simulink model "raibert_controller_1_2"  (R2018b)
settings: Solver=FixedStepDiscrete  StartTime=0.0  StopTime=inf  FixedStep=sample_time  RelTol=1e-3
InitFcn:
  | raibert_controller_params_1_2
  | warning off all
values from neighbouring files (symbols this model uses):
  sample_time = 1/sample_freq    (= 0.001)    [simulation_params.m]
undefined symbols (not defined in the file or in its folder): ctrl, Discrete, initial_dx_estimate, initial_dy_estimate, initial_dz_estimate, initial_z_estimate, Time
libraries: simulink x30, ctrlSharedLib x7
(part 2 of 4)

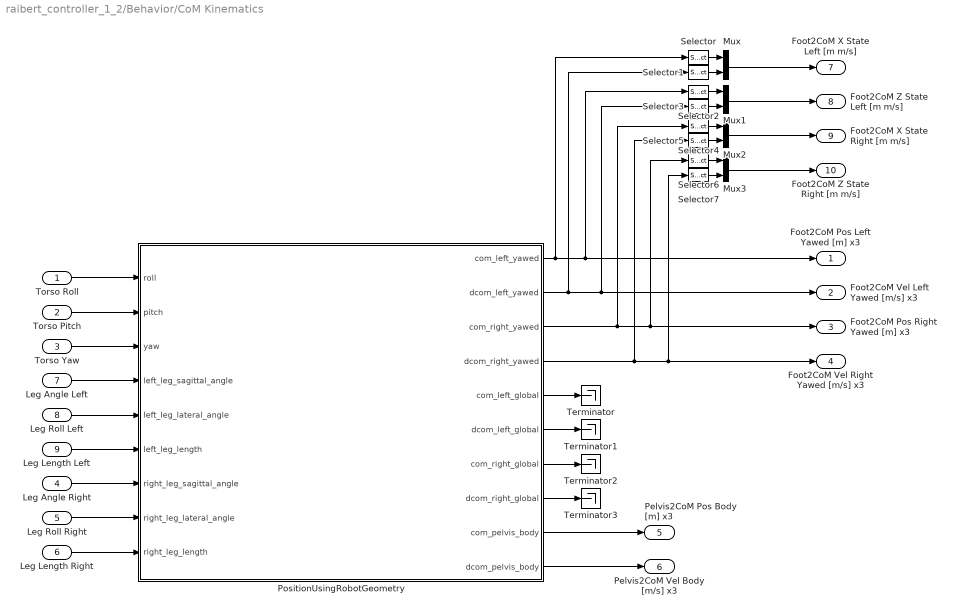
== system raibert_controller_1_2/Behavior/CoM Kinematics ==
  Torso Roll : Inport
  Torso Pitch : Inport  Port=2
  Torso Yaw : Inport  Port=3
  Leg Angle Right : Inport  Port=4
  Leg Roll Right : Inport  Port=5
  Leg Length Right : Inport  Port=6
  Leg Angle Left : Inport  Port=7
  Leg Roll Left : Inport  Port=8
  Leg Length Left : Inport  Port=9
  Mux{,1..3} (4 alike) : Mux  Inputs=2
  PositionUsingRobotGeometry : MATLAB Function  TreatAsAtomicUnit=on
  Selector{,1,4..5} (4 alike) : Selector  InputPortWidth=3  IndexOptions=Index vector (dialog)  Indices=[1]  OutputSizes=1
  Selector{2..3,6..7} (4 alike) : Selector  InputPortWidth=3  IndexOptions=Index vector (dialog)  Indices=[3]  OutputSizes=1
  Terminator{,1..3} (4 alike) : Terminator
  Foot2CoM Pos Left Yawed [m] x3 : Outport
  Foot2CoM Vel Left Yawed [m/s] x3 : Outport  Port=2
  Foot2CoM Pos Right Yawed [m] x3 : Outport  Port=3
  Foot2CoM Vel Right Yawed [m/s] x3 : Outport  Port=4
  Pelvis2CoM Pos Body [m] x3 : Outport  Port=5
  Pelvis2CoM Vel Body [m/s] x3 : Outport  Port=6
  Foot2CoM X State Left [m m/s] : Outport  Port=7
  Foot2CoM Z State Left [m m/s] : Outport  Port=8
  Foot2CoM X State Right [m m/s] : Outport  Port=9
  Foot2CoM Z State Right [m m/s] : Outport  Port=10
  wires:
  Leg Angle Left/1 -> PositionUsingRobotGeometry/4(left_leg_sagittal_angle)
  Leg Roll Left/1 -> PositionUsingRobotGeometry/5(left_leg_lateral_angle)
  Leg Length Left/1 -> PositionUsingRobotGeometry/6(left_leg_length)
  Leg Angle Right/1 -> PositionUsingRobotGeometry/7(right_leg_sagittal_angle)
  Leg Roll Right/1 -> PositionUsingRobotGeometry/8(right_leg_lateral_angle)
  Leg Length Right/1 -> PositionUsingRobotGeometry/9(right_leg_length)
  Torso Roll/1 -> PositionUsingRobotGeometry/1(roll)
  Torso Yaw/1 -> PositionUsingRobotGeometry/3(yaw)
  Torso Pitch/1 -> PositionUsingRobotGeometry/2(pitch)
  PositionUsingRobotGeometry/3(com_right_yawed) -> Selector4/1, Selector6/1, Foot2CoM Pos Right Yawed [m] x3/1
  PositionUsingRobotGeometry/4(dcom_right_yawed) -> Selector5/1, Selector7/1, Foot2CoM Vel Right Yawed [m/s] x3/1
  PositionUsingRobotGeometry/1(com_left_yawed) -> Foot2CoM Pos Left Yawed [m] x3/1, Selector2/1, Selector/1
  PositionUsingRobotGeometry/2(dcom_left_yawed) -> Selector3/1, Foot2CoM Vel Left Yawed [m/s] x3/1, Selector1/1
  PositionUsingRobotGeometry/10(dcom_pelvis_body) -> Pelvis2CoM Vel Body [m/s] x3/1
  PositionUsingRobotGeometry/9(com_pelvis_body) -> Pelvis2CoM Pos Body [m] x3/1
  PositionUsingRobotGeometry/5(com_left_global) -> Terminator/1
  PositionUsingRobotGeometry/6(dcom_left_global) -> Terminator1/1
  PositionUsingRobotGeometry/7(com_right_global) -> Terminator2/1
  PositionUsingRobotGeometry/8(dcom_right_global) -> Terminator3/1
  Selector/1 -> Mux/1
  Selector1/1 -> Mux/2
  Mux/1 -> Foot2CoM X State Left [m m/s]/1
  Selector3/1 -> Mux1/2
  Selector2/1 -> Mux1/1
  Mux1/1 -> Foot2CoM Z State Left [m m/s]/1
  Mux3/1 -> Foot2CoM Z State Right [m m/s]/1
  Selector6/1 -> Mux3/1
  Selector7/1 -> Mux3/2
  Mux2/1 -> Foot2CoM X State Right [m m/s]/1
  Selector5/1 -> Mux2/2
  Selector4/1 -> Mux2/1

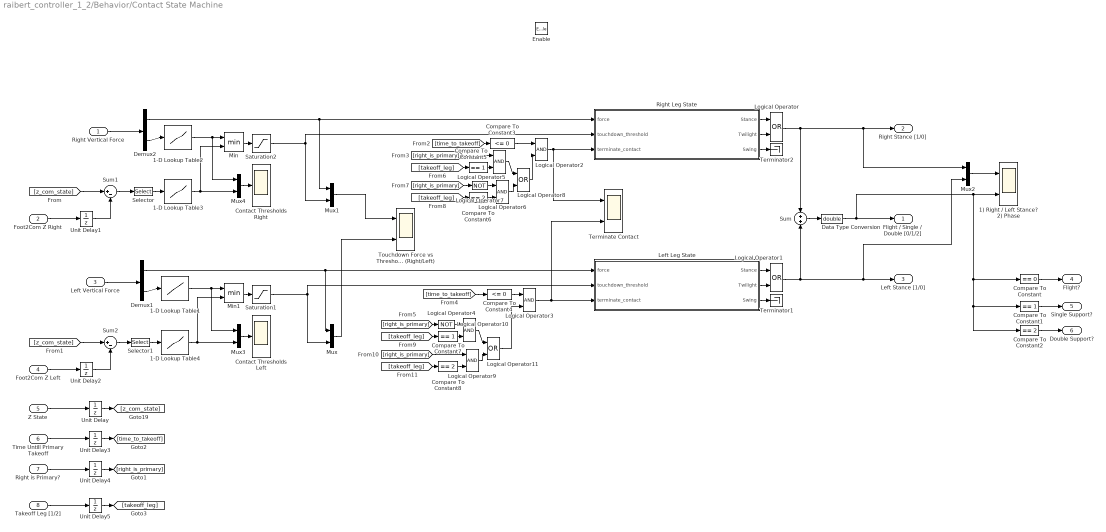
== system raibert_controller_1_2/Behavior/Contact State Machine ==
  Right Vertical Force : Inport
  Foot2Com Z Right : Inport  Port=2
  Left Vertical Force : Inport  Port=3
  Foot2Com Z Left : Inport  Port=4
  Z State : Inport  Port=5
  Time Untill Primary Takeoff : Inport  Port=6
  Right is Primary? : Inport  Port=7
  Takeoff Leg [1/2] : Inport  Port=8
  Enable : EnablePort  StatesWhenEnabling=reset
  1) Right / Left Stance? 2) Phase : Scope  NumInputPorts=2
  1-D Lookup Table1 : Lookup_n-D  NumberOfTableDimensions=1  BreakpointsForDimension1=[0, ctrl.touchdown_force_rate_hi]  Table=[ctrl.touchdown_threshold_hi, ctrl.touchdown_threshold_lo]  InternalRulePriority=Speed  RndMeth=Simplest  InputSameDT=on
  1-D Lookup Table2 : Lookup_n-D  NumberOfTableDimensions=1  BreakpointsForDimension1=[0, ctrl.touchdown_force_rate_hi]  Table=[ctrl.touchdown_threshold_hi, ctrl.touchdown_threshold_lo]  InternalRulePriority=Speed  RndMeth=Simplest  InputSameDT=on
  1-D Lookup Table3 : Lookup_n-D  NumberOfTableDimensions=1  BreakpointsForDimension1=[0, ctrl.touchdown_dist_hi]  Table=[ctrl.touchdown_threshold_lo, ctrl.touchdown_threshold_hi]  InternalRulePriority=Speed  RndMeth=Simplest  InputSameDT=on
  1-D Lookup Table4 : Lookup_n-D  NumberOfTableDimensions=1  BreakpointsForDimension1=[0, ctrl.touchdown_dist_hi]  Table=[ctrl.touchdown_threshold_lo, ctrl.touchdown_threshold_hi]  InternalRulePriority=Speed  RndMeth=Simplest  InputSameDT=on
  Compare To Constant : simulink/Logic and Bit Operations/Compare To Constant  relop===  const=0  OutDataTypeStr=boolean
  Compare To Constant1 : simulink/Logic and Bit Operations/Compare To Constant  relop===  const=1  OutDataTypeStr=boolean
  Compare To Constant2 : simulink/Logic and Bit Operations/Compare To Constant  relop===  const=2  OutDataTypeStr=boolean
  Compare To Constant3 : simulink/Logic and Bit Operations/Compare To Constant  relop=<=  const=0  OutDataTypeStr=boolean
  Compare To Constant4 : simulink/Logic and Bit Operations/Compare To Constant  relop=<=  const=0  OutDataTypeStr=boolean
  Compare To Constant5 : simulink/Logic and Bit Operations/Compare To Constant  relop===  const=1  OutDataTypeStr=boolean
  Compare To Constant6 : simulink/Logic and Bit Operations/Compare To Constant  relop===  const=2  OutDataTypeStr=boolean
  Compare To Constant7 : simulink/Logic and Bit Operations/Compare To Constant  relop===  const=1  OutDataTypeStr=boolean
  Compare To Constant8 : simulink/Logic and Bit Operations/Compare To Constant  relop===  const=2  OutDataTypeStr=boolean
  Contact Thresholds Left : Scope
  Contact Thresholds Right : Scope
  Data Type Conversion : DataTypeConversion  OutDataTypeStr=double
  Demux1 : Demux  Outputs=2
  Demux2 : Demux  Outputs=2
  Left Leg State : State Transition Table  TreatAsAtomicUnit=on
  Logical Operator{,1,8,11} (4 alike) : Logic  Operator=OR  AllPortsSameDT=off  OutDataTypeStr=boolean
  Logical Operator10 : Logic  Operator=NOT  AllPortsSameDT=off  OutDataTypeStr=boolean
  Logical Operator{2..6,9} (6 alike) : Logic  AllPortsSameDT=off  OutDataTypeStr=boolean
  Logical Operator7 : Logic  Operator=NOT  AllPortsSameDT=off  OutDataTypeStr=boolean
  Min : MinMax  Inputs=2
  Min1 : MinMax  Inputs=2
  Mux{,1..4} (5 alike) : Mux  Inputs=2
  Right Leg State : State Transition Table  TreatAsAtomicUnit=on
  Saturation1 : Saturate  UpperLimit=ctrl.touchdown_threshold_hi  LowerLimit=ctrl.touchdown_threshold_lo
  Saturation2 : Saturate  UpperLimit=ctrl.touchdown_threshold_hi  LowerLimit=ctrl.touchdown_threshold_lo
  Selector : Selector  InputPortWidth=2  IndexOptions=Index vector (dialog)  Indices=[1]  OutputSizes=1
  Selector1 : Selector  InputPortWidth=2  IndexOptions=Index vector (dialog)  Indices=[1]  OutputSizes=1
  Sum : Sum  Inputs=+|+
  Sum1 : Sum  Inputs=|+-
  Sum2 : Sum  Inputs=|+-
  Terminate Contact : Scope  NumInputPorts=2
  Terminator1 : Terminator
  Terminator2 : Terminator
  Touchdown Force vs Threshold (Right/Left) : Scope  NumInputPorts=2
  Unit Delay{,1..5} (6 alike) : UnitDelay  SampleTime=-1
  Flight / Single / Double [0/1/2] : Outport  InitialOutput=0
  Right Stance [1/0] : Outport  Port=2  InitialOutput=0
  Left Stance [1/0] : Outport  Port=3  InitialOutput=0
  Flight? : Outport  Port=4  InitialOutput=true
  Single Support? : Outport  Port=5  InitialOutput=false
  Double Support? : Outport  Port=6  InitialOutput=false
  wires:
  Left Leg State/3(" Swing") -> Terminator1/1
  Logical Operator/1 -> Sum/1, Mux2/1, Right Stance [1/0]/1
  Left Vertical Force/1 -> Demux1/1
  Demux1/2 -> 1-D Lookup Table1/1
  Demux1/1 -> Left Leg State/1(force), Mux/1
  Saturation1/1 -> Mux/2, Left Leg State/2(touchdown_threshold)
  Logical Operator1/1 -> Sum/2, Mux2/2, Left Stance [1/0]/1
  Mux/1 -> Touchdown Force vs Threshold (Right/Left)/2
  Mux1/1 -> Touchdown Force vs Threshold (Right/Left)/1
  Saturation2/1 -> Mux1/2, Right Leg State/2(touchdown_threshold)
  Demux2/1 -> Right Leg State/1(force), Mux1/1
  Demux2/2 -> 1-D Lookup Table2/1
  Right Vertical Force/1 -> Demux2/1
  Min/1 -> Saturation2/1
  Mux2/1 -> 1) Right / Left Stance? 2) Phase/1
  Sum/1 -> Data Type Conversion/1
  Compare To Constant/1 -> Flight?/1
  Compare To Constant1/1 -> Single Support?/1
  Compare To Constant2/1 -> Double Support?/1
  Data Type Conversion/1 -> Compare To Constant2/1, Compare To Constant1/1, Compare To Constant/1, 1) Right / Left Stance? 2) Phase/2, Flight / Single / Double [0/1/2]/1
  Right Leg State/3(" Swing") -> Terminator2/1
  Right Leg State/2(" Twilight") -> Logical Operator/2
  Right Leg State/1(" Stance") -> Logical Operator/1
  Left Leg State/1(" Stance") -> Logical Operator1/1
  Left Leg State/2(" Twilight") -> Logical Operator1/2
  Z State/1 -> Unit Delay/1
  [z_com_state] -> Sum1/1
  Foot2Com Z Right/1 -> Unit Delay1/1
  Foot2Com Z Left/1 -> Unit Delay2/1
  [z_com_state] -> Sum2/1
  Sum1/1 -> Selector/1
  1-D Lookup Table2/1 -> Mux4/1, Min/1
  1-D Lookup Table3/1 -> Mux4/2, Min/2
  Sum2/1 -> Selector1/1
  1-D Lookup Table1/1 -> Mux3/1, Min1/1
  1-D Lookup Table4/1 -> Min1/2, Mux3/2
  Min1/1 -> Saturation1/1
  Mux3/1 -> Contact Thresholds Left/1
  Mux4/1 -> Contact Thresholds Right/1
  Selector/1 -> 1-D Lookup Table3/1
  Selector1/1 -> 1-D Lookup Table4/1
  Unit Delay/1 -> [z_com_state]
  Unit Delay1/1 -> Sum1/2
  Unit Delay2/1 -> Sum2/2
  Right is Primary?/1 -> Unit Delay4/1
  Time Untill Primary Takeoff/1 -> Unit Delay3/1
  [time_to_takeoff] -> Compare To Constant3/1
  Compare To Constant3/1 -> Logical Operator2/1
  [right_is_primary] -> Logical Operator5/1
  Logical Operator2/1 -> Terminate Contact/1, Right Leg State/3(terminate_contact)
  Unit Delay3/1 -> [time_to_takeoff]
  Unit Delay4/1 -> [right_is_primary]
  Compare To Constant4/1 -> Logical Operator3/1
  [time_to_takeoff] -> Compare To Constant4/1
  Logical Operator3/1 -> Left Leg State/3(terminate_contact), Terminate Contact/2
  Takeoff Leg [1/2]/1 -> Unit Delay5/1
  Unit Delay5/1 -> [takeoff_leg]
  [takeoff_leg] -> Compare To Constant5/1
  Compare To Constant5/1 -> Logical Operator5/2
  Compare To Constant6/1 -> Logical Operator6/2
  [takeoff_leg] -> Compare To Constant6/1
  [right_is_primary] -> Logical Operator7/1
  Logical Operator7/1 -> Logical Operator6/1
  Logical Operator5/1 -> Logical Operator8/1
  Logical Operator6/1 -> Logical Operator8/2
  Logical Operator8/1 -> Logical Operator2/2
  [right_is_primary] -> Logical Operator10/1
  Compare To Constant7/1 -> Logical Operator4/2
  Logical Operator4/1 -> Logical Operator11/1
  [takeoff_leg] -> Compare To Constant7/1
  Logical Operator9/1 -> Logical Operator11/2
  [right_is_primary] -> Logical Operator9/1
  Compare To Constant8/1 -> Logical Operator9/2
  [takeoff_leg] -> Compare To Constant8/1
  Logical Operator10/1 -> Logical Operator4/1
  Logical Operator11/1 -> Logical Operator3/2

== system raibert_controller_1_2/Behavior/Filter Gyro Velocities ==
  raw dq : Inport
  Demux : Demux  Outputs=3
  Demux1 : Demux  Outputs=3
  Fourbar : Selector  InputPortWidth=13  IndexOptions=Index vector (dialog)  Indices=[1 2 3 4 5 6 7 8]  OutputSizes=1
  IMU Two Pole Filter : DiscreteTransferFcn  Numerator=[ctrl.A_imu 0 0]  Denominator=[1 ctrl.B1_imu ctrl.B2_imu]  SampleTime=sample_time
  Lateral : Selector  InputPortWidth=13  IndexOptions=Index vector (dialog)  Indices=[9 10]  OutputSizes=1
  Mux : Mux  Inputs=3
  Mux25 : Mux  Inputs=2
  Mux26 : Mux  Inputs=2
  Mux27 : Mux  Inputs=2
  Torso Orientation : Selector  InputPortWidth=13  IndexOptions=Index vector (dialog)  Indices=[11 12 13]  OutputSizes=1
  Torso Orientation Filter : Scope  NumInputPorts=3
  filtered dq : Outport
  wires:
  Fourbar/1 -> Mux/1
  IMU Two Pole Filter/1 -> Demux1/1, Mux/3
  Mux/1 -> filtered dq/1
  raw dq/1 -> Fourbar/1, Torso Orientation/1, Lateral/1
  Torso Orientation/1 -> Demux/1, IMU Two Pole Filter/1
  Lateral/1 -> Mux/2
  Mux25/1 -> Torso Orientation Filter/1
  Mux27/1 -> Torso Orientation Filter/3
  Mux26/1 -> Torso Orientation Filter/2
  Demux/1 -> Mux25/1
  Demux/2 -> Mux26/1
  Demux/3 -> Mux27/1
  Demux1/1 -> Mux25/2
  Demux1/2 -> Mux26/2
  Demux1/3 -> Mux27/2

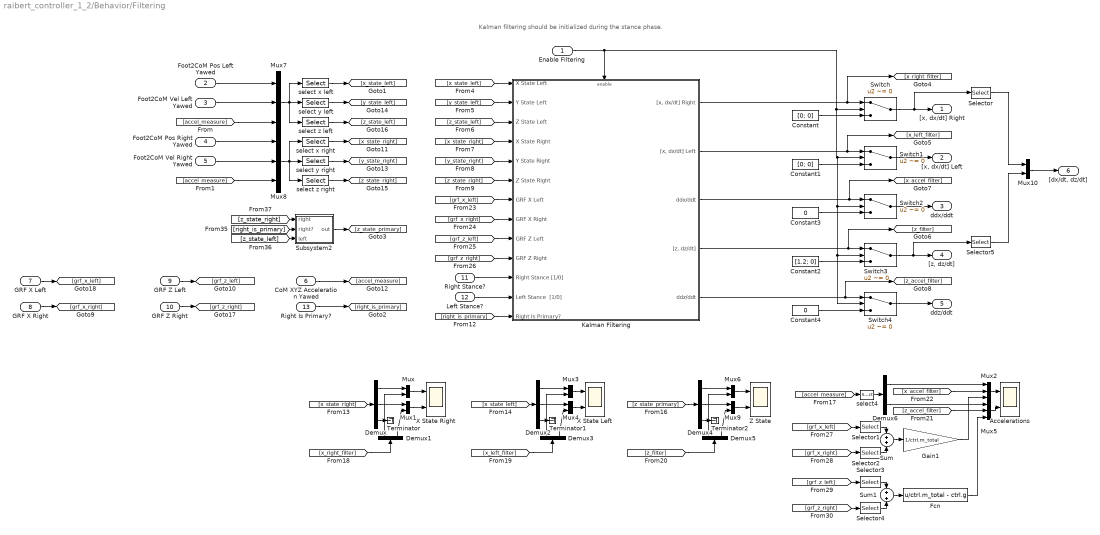
== system raibert_controller_1_2/Behavior/Filtering ==
  note: Kalman filtering should be initialized during the stance phase.
  Enable Filtering : Inport
  Foot2CoM Pos Left Yawed : Inport  Port=2
  Foot2CoM Vel Left Yawed : Inport  Port=3
  Foot2CoM Pos Right Yawed : Inport  Port=4
  Foot2CoM Vel Right Yawed : Inport  Port=5
  CoM XYZ Acceleration Yawed : Inport  Port=6
  GRF X Left : Inport  Port=7
  GRF X Right : Inport  Port=8
  GRF Z Left : Inport  Port=9
  GRF Z Right : Inport  Port=10
  Right Stance? : Inport  Port=11
  Left Stance? : Inport  Port=12
  Right Is Primary? : Inport  Port=13
  Accelerations : Scope  NumInputPorts=2
  Constant : Constant  Value=[0; 0]
  Constant1 : Constant  Value=[0; 0]
  Constant2 : Constant  Value=[1.2; 0]
  Constant3 : Constant  Value=0
  Constant4 : Constant  Value=0
  Demux : Demux  Outputs=3
  Demux{1,3,5..6} (4 alike) : Demux  Outputs=2
  Demux2 : Demux  Outputs=3
  Demux4 : Demux  Outputs=3
  Fcn : Fcn  Expr=u/ctrl.m_total - ctrl.g
  Gain1 : Gain  Gain=1/ctrl.m_total
  Kalman Filtering : Subsystem
  Mux{,1,3..4,6,9..10} (7 alike) : Mux  Inputs=2
  Mux{2,5,7..8} (4 alike) : Mux  Inputs=3
  Selector : Selector  InputPortWidth=2  IndexOptions=Index vector (dialog)  Indices=[2]  OutputSizes=1
  Selector{1..4} (4 alike) : Selector  InputPortWidth=2  IndexOptions=Index vector (dialog)  Indices=[1]  OutputSizes=1
  Selector5 : Selector  InputPortWidth=2  IndexOptions=Index vector (dialog)  Indices=[2]  OutputSizes=1
  Subsystem2 : Subsystem
  Sum : Sum  Inputs=+|+
  Sum1 : Sum  Inputs=+|+
  Switch{,1..4} (5 alike) : Switch  Criteria=u2 ~= 0
  Terminator : Terminator
  Terminator1 : Terminator
  Terminator2 : Terminator
  X State Left : Scope  NumInputPorts=2
  X State Right : Scope  NumInputPorts=2
  Z State : Scope  NumInputPorts=2
  select x left : Selector  InputPortWidth=9  IndexOptions=Index vector (dialog)  Indices=[1 4 7]  OutputSizes=1
  select x right : Selector  InputPortWidth=9  IndexOptions=Index vector (dialog)  Indices=[1 4 7]  OutputSizes=1
  select y left : Selector  InputPortWidth=9  IndexOptions=Index vector (dialog)  Indices=[2 5 8]  OutputSizes=1
  select y right : Selector  InputPortWidth=9  IndexOptions=Index vector (dialog)  Indices=[2 5 8]  OutputSizes=1
  select z left : Selector  InputPortWidth=9  IndexOptions=Index vector (dialog)  Indices=[3 6 9]  OutputSizes=1
  select z right : Selector  InputPortWidth=9  IndexOptions=Index vector (dialog)  Indices=[3 6 9]  OutputSizes=1
  select4 : Selector  InputPortWidth=3  IndexOptions=Index vector (dialog)  Indices=[1 3]  OutputSizes=1
  "[x, dx/dt] Right" : Outport
  "[x, dx/dt] Left" : Outport  Port=2
  ddx/ddt : Outport  Port=3
  "[z, dz/dt]" : Outport  Port=4
  ddz/ddt : Outport  Port=5
  "[dx/dt, dz/dt]" : Outport  Port=6
  wires:
  [grf_x_right] -> Kalman Filtering/8(GRF X Right)
  [grf_x_left] -> Kalman Filtering/7(GRF X Left)
  [grf_z_right] -> Kalman Filtering/10(GRF Z Right)
  Right Stance?/1 -> Kalman Filtering/11(Right Stance [1/0])
  [right_is_primary] -> Kalman Filtering/13(Right Is Primary?)
  [grf_z_left] -> Kalman Filtering/9(GRF Z Left)
  Enable Filtering/1 -> Switch4/2, Switch3/2, Switch2/2, Switch1/2, Switch/2, Kalman Filtering/Enable
  Left Stance?/1 -> Kalman Filtering/12(Left Stance  [1/0])
  Mux8/1 -> select z right/1, select y right/1, select x right/1
  Mux7/1 -> select z left/1, select y left/1, select x left/1
  Foot2CoM Vel Right Yawed/1 -> Mux8/2
  Foot2CoM Vel Left Yawed/1 -> Mux7/2
  Foot2CoM Pos Right Yawed/1 -> Mux8/1
  Kalman Filtering/1("[x, dx/dt] Right") -> [x_right_filter], Switch/1
  Kalman Filtering/2("[x, dx/dt] Left") -> [x_left_filter], Switch1/1
  Kalman Filtering/3(ddx/ddt) -> [x_accel_filter], Switch2/1
  Kalman Filtering/4("[z, dz/dt]") -> [z_filter], Switch3/1
  Kalman Filtering/5(ddz/ddt) -> [z_accel_filter], Switch4/1
  Switch/1 -> Selector/1, "[x, dx/dt] Right"/1
  Switch1/1 -> "[x, dx/dt] Left"/1
  Switch2/1 -> ddx/ddt/1
  Switch3/1 -> Selector5/1, "[z, dz/dt]"/1
  Switch4/1 -> ddz/ddt/1
  CoM XYZ Acceleration Yawed/1 -> [accel_measure]
  [accel_measure] -> Mux7/3
  [accel_measure] -> Mux8/3
  Constant3/1 -> Switch2/3
  Constant4/1 -> Switch4/3
  select x left/1 -> [x_state_left]
  select y left/1 -> [y_state_left]
  select z left/1 -> [z_state_left]
  select z right/1 -> [z_state_right]
  select y right/1 -> [y_state_right]
  select x right/1 -> [x_state_right]
  [z_state_right] -> Kalman Filtering/6(Z State Right)
  [y_state_right] -> Kalman Filtering/5(Y State Right)
  [x_state_right] -> Kalman Filtering/4(X State Right)
  [z_state_left] -> Kalman Filtering/3(Z State Left)
  [y_state_left] -> Kalman Filtering/2(Y State Left)
  [x_state_left] -> Kalman Filtering/1(X State Left)
  [right_is_primary] -> Subsystem2/2(right?)
  Right Is Primary?/1 -> [right_is_primary]
  Constant/1 -> Switch/3
  Constant1/1 -> Switch1/3
  [z_state_left] -> Subsystem2/3(left)
  [z_state_right] -> Subsystem2/1(right)
  Mux/1 -> X State Right/1
  Mux1/1 -> X State Right/2
  [x_state_right] -> Demux/1
  Demux/1 -> Mux/1
  Demux/2 -> Mux1/1
  Demux1/1 -> Mux/2
  Demux1/2 -> Mux1/2
  Demux3/2 -> Mux4/2
  Demux3/1 -> Mux3/2
  Demux2/2 -> Mux4/1
  Demux2/1 -> Mux3/1
  [x_state_left] -> Demux2/1
  Mux4/1 -> X State Left/2
  Mux3/1 -> X State Left/1
  Mux6/1 -> Z State/1
  Mux9/1 -> Z State/2
  Constant2/1 -> Switch3/3
  Demux4/1 -> Mux6/1
  Demux4/2 -> Mux9/1
  Demux5/1 -> Mux6/2
  Demux5/2 -> Mux9/2
  Demux/3 -> Terminator/1
  Demux2/3 -> Terminator1/1
  Demux4/3 -> Terminator2/1
  Subsystem2/1(out) -> [z_state_primary]
  [z_state_primary] -> Demux4/1
  Foot2CoM Pos Left Yawed/1 -> Mux7/1
  Mux5/1 -> Accelerations/2
  Mux2/1 -> Accelerations/1
  [x_right_filter] -> Demux1/1
  [x_left_filter] -> Demux3/1
  [z_filter] -> Demux5/1
  [accel_measure] -> select4/1
  Demux6/1 -> Mux2/1
  Demux6/2 -> Mux5/1
  [x_accel_filter] -> Mux2/2
  [z_accel_filter] -> Mux5/2
  select4/1 -> Demux6/1
  GRF X Left/1 -> [grf_x_left]
  GRF X Right/1 -> [grf_x_right]
  GRF Z Left/1 -> [grf_z_left]
  GRF Z Right/1 -> [grf_z_right]
  Selector1/1 -> Sum/1
  Selector2/1 -> Sum/2
  [grf_x_left] -> Selector1/1
  [grf_x_right] -> Selector2/1
  Selector4/1 -> Sum1/2
  Selector3/1 -> Sum1/1
  [grf_z_left] -> Selector3/1
  [grf_z_right] -> Selector4/1
  Sum/1 -> Gain1/1
  Sum1/1 -> Fcn/1
  Gain1/1 -> Mux2/3
  Fcn/1 -> Mux5/3
  Mux10/1 -> "[dx/dt, dz/dt]"/1
  Selector/1 -> Mux10/1
  Selector5/1 -> Mux10/2

== system raibert_controller_1_2/Behavior/L Leg Calculator ==
  Front [rad rad/s] : Inport
  Back [rad rad/s] : Inport  Port=2
  Demux1 : Demux  Outputs=2
  Gain1 : Gain  Gain=2*ctrl.l_seg
  Gain2 : Gain  Gain=ctrl.l_seg
  Gain4 : Gain  Gain=0.5
  Gain5 : Gain  Gain=0.5
  Gain7 : Gain  Gain=-ctrl.l_seg
  Gain8 : Gain  Gain=2*ctrl.l_seg
  Mux1 : Mux  Inputs=2
  Mux2 : Mux  Inputs=2
  Product2 : Product  RndMeth=Zero
  Product3 : Product  RndMeth=Zero
  Sum4 : Sum  Inputs=+|+
  Sum5 : Sum  Inputs=+|-
  Trigonometric Function : Trigonometry  Operator=cos
  Trigonometric Function1 : Trigonometry
  Trigonometric Function2 : Trigonometry  Operator=cos
  Trigonometric Function3 : Trigonometry
  "Leg Length [m m/s] " : Outport
  Leg Angle [rad rad/s] : Outport  Port=2
  Leg Splay [rad rad/s] : Outport  Port=3
  Leg Width [m m/s] : Outport  Port=4
  wires:
  Demux1/2 -> Product3/2, Product2/2
  Product3/1 -> Mux1/2  "leg length velocity"
  Product2/1 -> Mux2/2  "leg width velocity"
  Gain7/1 -> Product3/1
  Gain2/1 -> Product2/1
  Trigonometric Function3/1 -> Gain7/1
  Gain8/1 -> Mux2/1  "leg width position"
  Trigonometric Function1/1 -> Gain8/1
  Gain1/1 -> Mux1/1  "leg length position"
  Gain4/1 -> Trigonometric Function1/1, Trigonometric Function/1, Trigonometric Function3/1, Trigonometric Function2/1
  Mux2/1 -> Leg Width [m m/s]/1
  Trigonometric Function/1 -> Gain1/1
  Trigonometric Function2/1 -> Gain2/1
  Front [rad rad/s]/1 -> Sum4/2, Sum5/2
  Back [rad rad/s]/1 -> Sum4/1, Sum5/1
  Demux1/1 -> Gain4/1
  Sum5/1 -> Leg Splay [rad rad/s]/1, Demux1/1
  Mux1/1 -> "Leg Length [m m/s] "/1
  Sum4/1 -> Gain5/1
  Gain5/1 -> Leg Angle [rad rad/s]/1

== system raibert_controller_1_2/Behavior/Latch ==
  Enable : EnablePort
  Constant : Constant  Value=true
  latched : Outport  InitialOutput=false
  wires:
  Constant/1 -> latched/1

== system raibert_controller_1_2/Behavior/Latch3 ==
  Enable : EnablePort
  Constant : Constant  Value=true
  latched : Outport  InitialOutput=false
  wires:
  Constant/1 -> latched/1

== system raibert_controller_1_2/Behavior/Leg Plane GRF Left ==
  Leg Angle : Inport  PortDimensions=2
  Torso Pitch : Inport  Port=2  PortDimensions=2
  Axial React Force : Inport  Port=3  PortDimensions=2
  Ortho React Force : Inport  Port=4  PortDimensions=2
  World Frame React Forces : MATLAB Function  TreatAsAtomicUnit=on
  Horizontal Force : Outport  PortDimensions=2
  Vertical Force : Outport  Port=2  PortDimensions=2
  wires:
  Ortho React Force/1 -> World Frame React Forces/4(F_ortho)
  Axial React Force/1 -> World Frame React Forces/3(F_axial)
  Torso Pitch/1 -> World Frame React Forces/2(torso_pitch)
  Leg Angle/1 -> World Frame React Forces/1(leg_angle)
  World Frame React Forces/2(F_vert) -> Vertical Force/1
  World Frame React Forces/1(F_horz) -> Horizontal Force/1

== system raibert_controller_1_2/Behavior/Leg Plane GRF Right ==
  Leg Angle : Inport  PortDimensions=2
  Torso Pitch : Inport  Port=2  PortDimensions=2
  Axial React Force : Inport  Port=3  PortDimensions=2
  Ortho React Force : Inport  Port=4  PortDimensions=2
  World Frame React Forces : MATLAB Function  TreatAsAtomicUnit=on
  Horizontal Force : Outport  PortDimensions=2
  Vertical Force : Outport  Port=2  PortDimensions=2
  wires:
  Leg Angle/1 -> World Frame React Forces/1(leg_angle)
  Torso Pitch/1 -> World Frame React Forces/2(torso_pitch)
  Axial React Force/1 -> World Frame React Forces/3(F_axial)
  Ortho React Force/1 -> World Frame React Forces/4(F_ortho)
  World Frame React Forces/1(F_horz) -> Horizontal Force/1
  World Frame React Forces/2(F_vert) -> Vertical Force/1

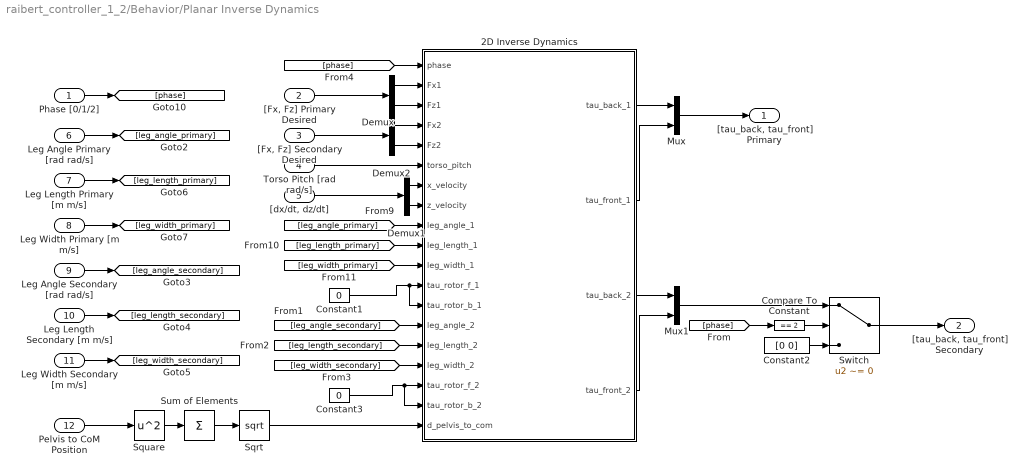
== system raibert_controller_1_2/Behavior/Planar Inverse Dynamics ==
  Phase [0/1/2] : Inport
  "[Fx, Fz] Primary Desired" : Inport  Port=2
  "[Fx, Fz] Secondary Desired" : Inport  Port=3
  Torso Pitch [rad rad/s] : Inport  Port=4
  "[dx/dt, dz/dt]" : Inport  Port=5
  Leg Angle Primary [rad rad/s] : Inport  Port=6
  Leg Length Primary [m m/s] : Inport  Port=7
  Leg Width Primary [m m/s] : Inport  Port=8
  Leg Angle Secondary [rad rad/s] : Inport  Port=9
  Leg Length Secondary [m m/s] : Inport  Port=10
  Leg Width Secondary [m m/s] : Inport  Port=11
  Pelvis to CoM Position : Inport  Port=12
  2D Inverse Dynamics : MATLAB Function  TreatAsAtomicUnit=on
  Compare To Constant : simulink/Logic and Bit Operations/Compare To Constant  relop===  const=2  OutDataTypeStr=boolean
  Constant1 : Constant  Value=0
  Constant2 : Constant  Value=[0 0]
  Constant3 : Constant  Value=0
  Demux : Demux  Outputs=2
  Demux1 : Demux  Outputs=2
  Demux2 : Demux  Outputs=2
  Mux : Mux  Inputs=2
  Mux1 : Mux  Inputs=2
  Sqrt : Sqrt  SaturateOnIntegerOverflow=on
  Square : Math  Operator=square  SaturateOnIntegerOverflow=on
  Sum of Elements : Sum  Inputs=+
  Switch : Switch  Criteria=u2 ~= 0
  "[tau_back, tau_front] Primary" : Outport
  "[tau_back, tau_front] Secondary" : Outport  Port=2
  wires:
  Mux/1 -> "[tau_back, tau_front] Primary"/1
  Pelvis to CoM Position/1 -> Square/1
  Square/1 -> Sum of Elements/1
  Sum of Elements/1 -> Sqrt/1
  "[Fx, Fz] Primary Desired"/1 -> Demux/1
  Leg Angle Primary [rad rad/s]/1 -> [leg_angle_primary]
  Leg Angle Secondary [rad rad/s]/1 -> [leg_angle_secondary]
  Leg Length Secondary [m m/s]/1 -> [leg_length_secondary]
  Leg Width Secondary [m m/s]/1 -> [leg_width_secondary]
  Leg Width Primary [m m/s]/1 -> [leg_width_primary]
  Leg Length Primary [m m/s]/1 -> [leg_length_primary]
  Phase [0/1/2]/1 -> [phase]
  2D Inverse Dynamics/1(tau_back_1) -> Mux/1
  2D Inverse Dynamics/2(tau_front_1) -> Mux/2
  Demux/1 -> 2D Inverse Dynamics/2(Fx1)
  Demux/2 -> 2D Inverse Dynamics/3(Fz1)
  Torso Pitch [rad rad/s]/1 -> 2D Inverse Dynamics/6(torso_pitch)
  [leg_angle_primary] -> 2D Inverse Dynamics/9(leg_angle_1)
  [leg_length_primary] -> 2D Inverse Dynamics/10(leg_length_1)
  [leg_width_primary] -> 2D Inverse Dynamics/11(leg_width_1)
  [leg_angle_secondary] -> 2D Inverse Dynamics/14(leg_angle_2)
  [leg_width_secondary] -> 2D Inverse Dynamics/16(leg_width_2)
  [leg_length_secondary] -> 2D Inverse Dynamics/15(leg_length_2)
  Constant1/1 -> 2D Inverse Dynamics/12(tau_rotor_f_1), 2D Inverse Dynamics/13(tau_rotor_b_1)
  Constant3/1 -> 2D Inverse Dynamics/17(tau_rotor_f_2), 2D Inverse Dynamics/18(tau_rotor_b_2)
  2D Inverse Dynamics/3(tau_back_2) -> Mux1/1
  2D Inverse Dynamics/4(tau_front_2) -> Mux1/2
  "[dx/dt, dz/dt]"/1 -> Demux1/1
  Demux1/2 -> 2D Inverse Dynamics/8(z_velocity)
  Demux1/1 -> 2D Inverse Dynamics/7(x_velocity)
  Demux2/1 -> 2D Inverse Dynamics/4(Fx2)
  Demux2/2 -> 2D Inverse Dynamics/5(Fz2)
  "[Fx, Fz] Secondary Desired"/1 -> Demux2/1
  [phase] -> Compare To Constant/1
  Constant2/1 -> Switch/3
  Mux1/1 -> Switch/1
  Compare To Constant/1 -> Switch/2
  Switch/1 -> "[tau_back, tau_front] Secondary"/1
  [phase] -> 2D Inverse Dynamics/1(phase)
  Sqrt/1 -> 2D Inverse Dynamics/19(d_pelvis_to_com)

== system raibert_controller_1_2/Behavior/R Leg Calculator ==
  Front [rad rad/s] : Inport
  Back [rad rad/s] : Inport  Port=2
  Demux1 : Demux  Outputs=2
  Gain1 : Gain  Gain=2*ctrl.l_seg
  Gain2 : Gain  Gain=ctrl.l_seg
  Gain4 : Gain  Gain=0.5
  Gain5 : Gain  Gain=0.5
  Gain7 : Gain  Gain=-ctrl.l_seg
  Gain8 : Gain  Gain=2*ctrl.l_seg
  Mux1 : Mux  Inputs=2
  Mux2 : Mux  Inputs=2
  Product2 : Product  RndMeth=Zero
  Product3 : Product  RndMeth=Zero
  Sum4 : Sum  Inputs=+|+
  Sum5 : Sum  Inputs=+|-
  Trigonometric Function : Trigonometry  Operator=cos
  Trigonometric Function1 : Trigonometry
  Trigonometric Function2 : Trigonometry  Operator=cos
  Trigonometric Function3 : Trigonometry
  "Leg Length [m m/s] " : Outport
  Leg Angle [rad rad/s] : Outport  Port=2
  Leg Splay [rad rad/s] : Outport  Port=3
  Leg Width [m m/s] : Outport  Port=4
  wires:
  Gain5/1 -> Leg Angle [rad rad/s]/1
  Sum4/1 -> Gain5/1
  Mux1/1 -> "Leg Length [m m/s] "/1
  Sum5/1 -> Demux1/1, Leg Splay [rad rad/s]/1
  Demux1/1 -> Gain4/1
  Back [rad rad/s]/1 -> Sum5/1, Sum4/1
  Front [rad rad/s]/1 -> Sum5/2, Sum4/2
  Trigonometric Function2/1 -> Gain2/1
  Trigonometric Function/1 -> Gain1/1
  Mux2/1 -> Leg Width [m m/s]/1
  Gain4/1 -> Trigonometric Function2/1, Trigonometric Function3/1, Trigonometric Function/1, Trigonometric Function1/1
  Gain1/1 -> Mux1/1  "leg length position"
  Trigonometric Function1/1 -> Gain8/1
  Gain8/1 -> Mux2/1  "leg width position"
  Trigonometric Function3/1 -> Gain7/1
  Gain2/1 -> Product2/1
  Gain7/1 -> Product3/1
  Product2/1 -> Mux2/2  "leg width velocity"
  Product3/1 -> Mux1/2  "leg length velocity"
  Demux1/2 -> Product2/2, Product3/2

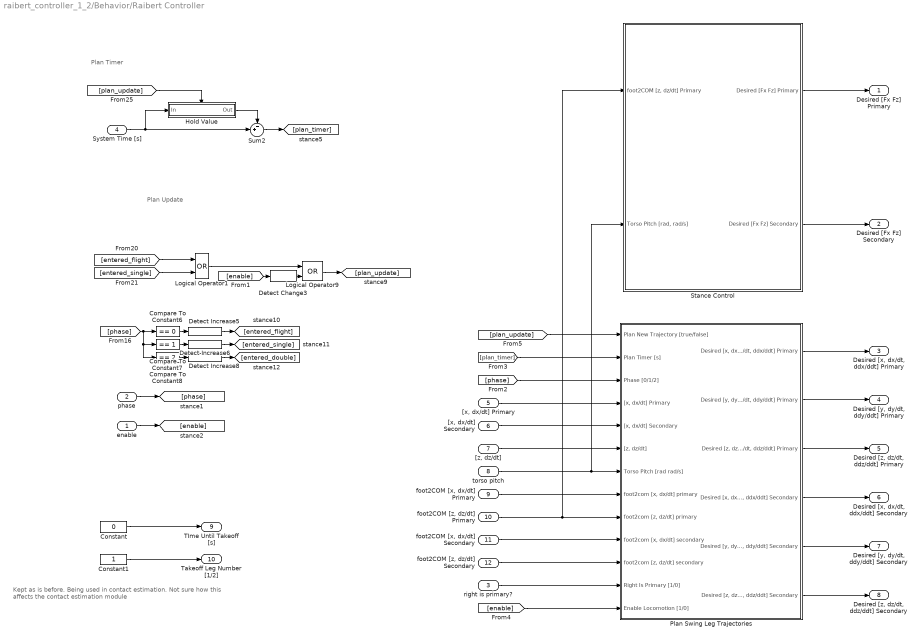
== system raibert_controller_1_2/Behavior/Raibert Controller ==
  note: Kept as is before. Being used in contact estimation.
      | Not sure how this affects the contact estimation module
  note: Plan Timer
  note: Plan Update
  enable : Inport
  phase : Inport  Port=2
  right is primary? : Inport  Port=3
  System Time [s] : Inport  Port=4
  "[x, dx/dt] Primary" : Inport  Port=5
  "[x, dx/dt] Secondary" : Inport  Port=6
  "[z, dz/dt]" : Inport  Port=7
  torso pitch : Inport  Port=8
  "foot2COM [x, dx/dt] Primary" : Inport  Port=9
  "foot2COM [z, dz/dt] Primary" : Inport  Port=10
  "foot2COM [x, dx/dt] Secondary" : Inport  Port=11
  "foot2COM [z, dz/dt] Secondary" : Inport  Port=12
  Compare To Constant6 : simulink/Logic and Bit Operations/Compare To Constant  relop===  const=0  OutDataTypeStr=boolean
  Compare To Constant7 : simulink/Logic and Bit Operations/Compare To Constant  relop===  const=1  OutDataTypeStr=boolean
  Compare To Constant8 : simulink/Logic and Bit Operations/Compare To Constant  relop===  const=2  OutDataTypeStr=boolean
  Constant : Constant  Value=0
  Constant1 : Constant
  Detect Change3 : simulink/Logic and Bit Operations/Detect Change  vinit=0  OutDataTypeStr=boolean
  Detect Increase5 : simulink/Logic and Bit Operations/Detect Increase  vinit=1  OutDataTypeStr=boolean
  Detect Increase6 : simulink/Logic and Bit Operations/Detect Increase  vinit=0.0  OutDataTypeStr=boolean
  Detect Increase8 : simulink/Logic and Bit Operations/Detect Increase  vinit=0.0  OutDataTypeStr=boolean
  Hold Value : Subsystem  TreatAsAtomicUnit=on
  Logical Operator1 : Logic  Operator=OR  AllPortsSameDT=off  OutDataTypeStr=boolean
  Logical Operator9 : Logic  Operator=OR  AllPortsSameDT=off  OutDataTypeStr=boolean
  Plan Swing Leg Trajectories : Subsystem
  Stance Control : Subsystem
  Sum2 : Sum  Inputs=-+|
  Desired [Fx Fz] Primary : Outport
  Desired [Fx Fz] Secondary : Outport  Port=2
  "Desired [x, dx/dt, ddx/ddt] Primary" : Outport  Port=3
  "Desired [y, dy/dt, ddy/ddt] Primary" : Outport  Port=4
  "Desired [z, dz/dt, ddz/ddt] Primary" : Outport  Port=5
  "Desired [x, dx/dt, ddx/ddt] Secondary" : Outport  Port=6
  "Desired [y, dy/dt, ddy/ddt] Secondary" : Outport  Port=7
  "Desired [z, dz/dt, ddz/ddt] Secondary" : Outport  Port=8
  TIme Until Takeoff [s] : Outport  Port=9
  Takeoff Leg Number [1/2] : Outport  Port=10
  wires:
  "[x, dx/dt] Primary"/1 -> Plan Swing Leg Trajectories/4("[x, dx/dt] Primary")
  Plan Swing Leg Trajectories/2("Desired [y, dy/dt, ddy/ddt] Primary") -> "Desired [y, dy/dt, ddy/ddt] Primary"/1
  Stance Control/2(Desired [Fx Fz] Secondary) -> Desired [Fx Fz] Secondary/1
  Plan Swing Leg Trajectories/6("Desired [z, dz/dt, ddz/ddt] Secondary") -> "Desired [z, dz/dt, ddz/ddt] Secondary"/1
  Plan Swing Leg Trajectories/5("Desired [y, dy/dt, ddy/ddt] Secondary") -> "Desired [y, dy/dt, ddy/ddt] Secondary"/1
  torso pitch/1 -> Stance Control/2("Torso Pitch [rad, rad/s]"), Plan Swing Leg Trajectories/7(Torso Pitch [rad rad/s])
  right is primary?/1 -> Plan Swing Leg Trajectories/12(Right Is Primary [1/0])
  Plan Swing Leg Trajectories/1("Desired [x, dx/dt, ddx/ddt] Primary") -> "Desired [x, dx/dt, ddx/ddt] Primary"/1
  Stance Control/1(Desired [Fx Fz] Primary) -> Desired [Fx Fz] Primary/1
  "[z, dz/dt]"/1 -> Plan Swing Leg Trajectories/6("[z, dz/dt]")
  "foot2COM [z, dz/dt] Primary"/1 -> Stance Control/1("foot2COM [z, dz/dt] Primary"), Plan Swing Leg Trajectories/9("foot2com [z, dz/dt] primary")
  "[x, dx/dt] Secondary"/1 -> Plan Swing Leg Trajectories/5("[x, dx/dt] Secondary")
  Plan Swing Leg Trajectories/3("Desired [z, dz/dt, ddz/ddt] Primary") -> "Desired [z, dz/dt, ddz/ddt] Primary"/1
  Plan Swing Leg Trajectories/4("Desired [x, dx/dt, ddx/ddt] Secondary") -> "Desired [x, dx/dt, ddx/ddt] Secondary"/1
  "foot2COM [x, dx/dt] Primary"/1 -> Plan Swing Leg Trajectories/8("foot2com [x, dx/dt] primary")
  [plan_update] -> Plan Swing Leg Trajectories/1(Plan New Trajectory [true/false])
  "foot2COM [z, dz/dt] Secondary"/1 -> Plan Swing Leg Trajectories/11("foot2com [z, dz/dt] secondary")
  "foot2COM [x, dx/dt] Secondary"/1 -> Plan Swing Leg Trajectories/10("foot2com [x, dx/dt] secondary")
  System Time [s]/1 -> Hold Value/1(In), Sum2/2
  Sum2/1 -> [plan_timer]
  [plan_update] -> Hold Value/Enable
  Hold Value/1(Out) -> Sum2/1
  Detect Change3/1 -> Logical Operator9/2
  Detect Increase6/1 -> [entered_single]
  Detect Increase8/1 -> [entered_double]
  [phase] -> Compare To Constant8/1, Compare To Constant7/1, Compare To Constant6/1
  [entered_single] -> Logical Operator1/2
  [enable] -> Detect Change3/1
  Compare To Constant6/1 -> Detect Increase5/1
  Logical Operator1/1 -> Logical Operator9/1
  Compare To Constant7/1 -> Detect Increase6/1
  [entered_flight] -> Logical Operator1/1
  Logical Operator9/1 -> [plan_update]
  Compare To Constant8/1 -> Detect Increase8/1
  Detect Increase5/1 -> [entered_flight]
  phase/1 -> [phase]
  [phase] -> Plan Swing Leg Trajectories/3(Phase [0/1/2])
  [plan_timer] -> Plan Swing Leg Trajectories/2(Plan Timer [s])
  enable/1 -> [enable]
  [enable] -> Plan Swing Leg Trajectories/13(Enable Locomotion [1/0])
  Constant/1 -> TIme Until Takeoff [s]/1
  Constant1/1 -> Takeoff Leg Number [1/2]/1

== system raibert_controller_1_2/Behavior/SEA Measurements ==
  Back Load Right : Inport  PortDimensions=2
  Back Motor Right : Inport  Port=2  PortDimensions=2
  Front Load Right : Inport  Port=3  PortDimensions=2
  Front Motor Right : Inport  Port=4  PortDimensions=2
  Back Load Left : Inport  Port=5  PortDimensions=2
  Back Motor Left : Inport  Port=6  PortDimensions=2
  Front Load Left : Inport  Port=7  PortDimensions=2
  Front Motor Left : Inport  Port=8  PortDimensions=2
  Leg Width Right : Inport  Port=9  PortDimensions=2
  Leg Length Right : Inport  Port=10  PortDimensions=2
  Leg Width Left : Inport  Port=11  PortDimensions=2
  Leg Length Left : Inport  Port=12  PortDimensions=2
  Gain : Gain  Gain=ctrl.k_sea(1)
  Gain1 : Gain  Gain=ctrl.k_sea(2)
  Gain2 : Gain  Gain=ctrl.k_sea(3)
  Gain3 : Gain  Gain=ctrl.k_sea(4)
  Leg Dynamics Left : MATLAB Function  TreatAsAtomicUnit=on
  Leg Dynamics Right : MATLAB Function  TreatAsAtomicUnit=on
  Sum{1..3,6} (4 alike) : Sum  Inputs=-+|
  Leg Axial React Force Right : Outport  PortDimensions=2
  Leg Ortho React Force Right : Outport  Port=2  PortDimensions=2
  Leg Axial React Force Left : Outport  Port=3  PortDimensions=2
  Leg Ortho React Force Left : Outport  Port=4  PortDimensions=2
  wires:
  Back Motor Right/1 -> Sum6/2
  Front Load Right/1 -> Sum1/1
  Front Motor Right/1 -> Sum1/2
  Back Load Right/1 -> Sum6/1
  Sum1/1 -> Gain1/1
  Sum6/1 -> Gain/1
  Back Motor Left/1 -> Sum2/2
  Front Load Left/1 -> Sum3/1
  Front Motor Left/1 -> Sum3/2
  Back Load Left/1 -> Sum2/1
  Sum2/1 -> Gain2/1
  Sum3/1 -> Gain3/1
  Leg Dynamics Right/1(axial_force) -> Leg Axial React Force Right/1
  Leg Dynamics Right/2(ortho_force) -> Leg Ortho React Force Right/1
  Leg Width Right/1 -> Leg Dynamics Right/3(leg_width)
  Leg Length Right/1 -> Leg Dynamics Right/4(leg_length)
  Leg Width Left/1 -> Leg Dynamics Left/3(leg_width)
  Leg Length Left/1 -> Leg Dynamics Left/4(leg_length)
  Leg Dynamics Left/2(ortho_force) -> Leg Ortho React Force Left/1
  Leg Dynamics Left/1(axial_force) -> Leg Axial React Force Left/1
  Gain/1 -> Leg Dynamics Right/1(tau_back)
  Gain1/1 -> Leg Dynamics Right/2(tau_front)
  Gain2/1 -> Leg Dynamics Left/1(tau_back)
  Gain3/1 -> Leg Dynamics Left/2(tau_front)

== system raibert_controller_1_2/Behavior/Select State Variables ==
  note: Order:
      |
      | backJointR
      | backGearR
      | frontJointR
      | fro ntGearR
      |
      | backJointL
      | backGearL
      | frontJointL
      | frontGearL
      |
      | latR
      | latL
      |
      | torsoRoll
      | torsoYaw
      | torsoPitch
  q : Inport
  dq/dt : Inport  Port=2
  Demux : Demux  Outputs=13
  Demux1 : Demux  Outputs=13
  Mux{,1..12} (13 alike) : Mux  Inputs=2
  back right load : Outport
  back right motor : Outport  Port=2
  front right load : Outport  Port=3
  front right motor : Outport  Port=4
  back left load : Outport  Port=5
  back left motor : Outport  Port=6
  front left load : Outport  Port=7
  front left motor : Outport  Port=8
  lateral right : Outport  Port=9
  lateral left : Outport  Port=10
  roll : Outport  Port=11
  yaw : Outport  Port=12
  pitch : Outport  Port=13
  wires:
  q/1 -> Demux/1
  dq/dt/1 -> Demux1/1
  Mux/1 -> back right load/1
  Mux1/1 -> back right motor/1
  Mux4/1 -> back left load/1
  Mux5/1 -> back left motor/1
  Mux8/1 -> lateral right/1
  Mux9/1 -> lateral left/1
  Mux12/1 -> pitch/1
  Mux2/1 -> front right load/1
  Mux3/1 -> front right motor/1
  Mux6/1 -> front left load/1
  Mux7/1 -> front left motor/1
  Mux10/1 -> roll/1
  Mux11/1 -> yaw/1
  Demux/1 -> Mux/1
  Demux1/1 -> Mux/2
  Demux/2 -> Mux1/1
  Demux/3 -> Mux2/1
  Demux/4 -> Mux3/1
  Demux/5 -> Mux4/1
  Demux/6 -> Mux5/1
  Demux/7 -> Mux6/1
  Demux/8 -> Mux7/1
  Demux/9 -> Mux8/1
  Demux/10 -> Mux9/1
  Demux/11 -> Mux10/1
  Demux/12 -> Mux11/1
  Demux/13 -> Mux12/1
  Demux1/2 -> Mux1/2
  Demux1/3 -> Mux2/2
  Demux1/4 -> Mux3/2
  Demux1/5 -> Mux4/2
  Demux1/6 -> Mux5/2
  Demux1/7 -> Mux6/2
  Demux1/8 -> Mux7/2
  Demux1/9 -> Mux8/2
  Demux1/10 -> Mux9/2
  Demux1/11 -> Mux10/2
  Demux1/12 -> Mux11/2
  Demux1/13 -> Mux12/2

== system raibert_controller_1_2/Behavior/Swing Control ==
  "foot2COM [z, dz/dt] Primary" : Inport
  "foot2COM [z, dz/dt] Secondary" : Inport  Port=2
  "foot2COM [x, dx/dt] Primary" : Inport  Port=3
  "foot2COM [x, dx/dt] Secondary" : Inport  Port=4
  Timer : Inport  Port=5
  Replan : Inport  Port=6
  Swing Trajectory Fit : MATLAB Function  TreatAsAtomicUnit=on
  Desired [x dx/dt ddx/ddt] Primary : Outport
  Desired [y dy/dt ddy/ddt] Primary : Outport  Port=2
  Desired [z dz/dt ddz/ddt] Primary : Outport  Port=3
  Desired [x dx/dt ddx/ddt] Secondary : Outport  Port=4
  Desired [y dy/dt ddy/ddt] Secondary : Outport  Port=5
  Desired [z dz/dt ddz/ddt] Secondary : Outport  Port=6

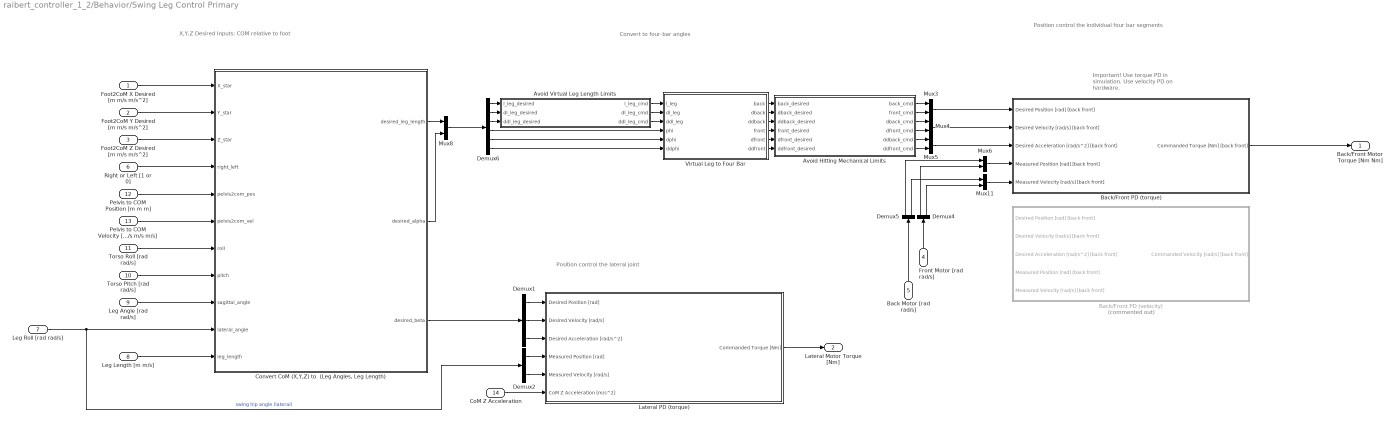
== system raibert_controller_1_2/Behavior/Swing Leg Control Primary ==
  note: Position control the lateral joint
  note: Important!
      | Use torque PD in simulation.
      | Use velocity PD on hardware.
  note: X,Y,Z Desired Inputs: COM relative to foot
  note: Convert to four-bar angles
  note: Position control the
      | individual four bar segments
  Foot2CoM X Desired [m m/s m/s^2] : Inport
  Foot2CoM Y Desired [m m/s m/s^2] : Inport  Port=2
  Foot2CoM Z Desired [m m/s m/s^2] : Inport  Port=3
  Front Motor [rad rad/s] : Inport  Port=4
  Back Motor [rad rad/s] : Inport  Port=5
  Right or Left [1 or 0] : Inport  Port=6
  Leg Roll [rad rad/s] : Inport  Port=7
  Leg Length [m m/s] : Inport  Port=8
  Leg Angle [rad rad/s] : Inport  Port=9
  Torso Pitch [rad rad/s] : Inport  Port=10
  Torso Roll [rad rad/s] : Inport  Port=11
  Pelvis to COM Position [m m m] : Inport  Port=12
  Pelvis to COM Velocity [m/s m/s m/s] : Inport  Port=13
  CoM Z Acceleration : Inport  Port=14
  Avoid Hitting Mechanical Limits : MATLAB Function  TreatAsAtomicUnit=on
  Avoid Virtual Leg Length Limits : MATLAB Function  TreatAsAtomicUnit=on
  Back/Front PD (torque) : Subsystem
  Back/Front PD (velocity) : Subsystem  Commented=on
  "Convert CoM (X,Y,Z) to  (Leg Angles, Leg Length)" : MATLAB Function  TreatAsAtomicUnit=on
  Demux1 : Demux  Outputs=3
  Demux2 : Demux  Outputs=2
  Demux4 : Demux  Outputs=2
  Demux5 : Demux  Outputs=2
  Demux6 : Demux  Outputs=6
  Lateral PD (torque) : Subsystem
  Mux{3..6,8,11} (6 alike) : Mux  Inputs=2
  Virtual Leg to Four Bar : MATLAB Function  TreatAsAtomicUnit=on
  Back/Front Motor Torque [Nm Nm] : Outport
  Lateral Motor Torque [Nm] : Outport  Port=2
  wires:
  CoM Z Acceleration/1 -> Lateral PD (torque)/6(CoM Z Acceleration [m/s^2])
  Demux2/1 -> Lateral PD (torque)/4(Measured Position [rad])
  Demux2/2 -> Lateral PD (torque)/5(Measured Velocity [rad/s])
  Lateral PD (torque)/1(Commanded Torque [Nm]) -> Lateral Motor Torque [Nm]/1
  Demux1/2 -> Lateral PD (torque)/2(Desired Velocity [rad/s])
  Demux1/3 -> Lateral PD (torque)/3(Desired Acceleration [rad/s^2])
  Demux1/1 -> Lateral PD (torque)/1(Desired Position [rad])
  Mux5/1 -> Back/Front PD (torque)/3(Desired Acceleration [rad/s^2] [back front])
  Demux6/3 -> Avoid Virtual Leg Length Limits/3(ddl_leg_desired)
  Demux6/2 -> Avoid Virtual Leg Length Limits/2(dl_leg_desired)
  Demux6/1 -> Avoid Virtual Leg Length Limits/1(l_leg_desired)
  Avoid Virtual Leg Length Limits/3(ddl_leg_cmd) -> Virtual Leg to Four Bar/3(ddl_leg)
  Avoid Virtual Leg Length Limits/2(dl_leg_cmd) -> Virtual Leg to Four Bar/2(dl_leg)
  Avoid Virtual Leg Length Limits/1(l_leg_cmd) -> Virtual Leg to Four Bar/1(l_leg)
  Foot2CoM X Desired [m m/s m/s^2]/1 -> "Convert CoM (X,Y,Z) to  (Leg Angles, Leg Length)"/1(X_star)
  Back/Front PD (torque)/1(Commanded Torque [Nm] [back front]) -> Back/Front Motor Torque [Nm Nm]/1
  "Convert CoM (X,Y,Z) to  (Leg Angles, Leg Length)"/3(desired_beta) -> Demux1/1
  Pelvis to COM Velocity [m/s m/s m/s]/1 -> "Convert CoM (X,Y,Z) to  (Leg Angles, Leg Length)"/6(pelvis2com_vel)
  Pelvis to COM Position [m m m]/1 -> "Convert CoM (X,Y,Z) to  (Leg Angles, Leg Length)"/5(pelvis2com_pos)
  Virtual Leg to Four Bar/5(dfront) -> Avoid Hitting Mechanical Limits/5(dfront_desired)
  Foot2CoM Y Desired [m m/s m/s^2]/1 -> "Convert CoM (X,Y,Z) to  (Leg Angles, Leg Length)"/2(Y_star)
  Mux8/1 -> Demux6/1
  "Convert CoM (X,Y,Z) to  (Leg Angles, Leg Length)"/1(desired_leg_length) -> Mux8/1
  Leg Length [m m/s]/1 -> "Convert CoM (X,Y,Z) to  (Leg Angles, Leg Length)"/11(leg_length)
  "Convert CoM (X,Y,Z) to  (Leg Angles, Leg Length)"/2(desired_alpha) -> Mux8/2
  Leg Angle [rad rad/s]/1 -> "Convert CoM (X,Y,Z) to  (Leg Angles, Leg Length)"/9(sagittal_angle)
  Leg Roll [rad rad/s]/1 -> "Convert CoM (X,Y,Z) to  (Leg Angles, Leg Length)"/10(lateral_angle), Demux2/1  "swing hip angle (lateral)"
  Right or Left [1 or 0]/1 -> "Convert CoM (X,Y,Z) to  (Leg Angles, Leg Length)"/4(right_left)
  Torso Roll [rad rad/s]/1 -> "Convert CoM (X,Y,Z) to  (Leg Angles, Leg Length)"/7(roll)
  Torso Pitch [rad rad/s]/1 -> "Convert CoM (X,Y,Z) to  (Leg Angles, Leg Length)"/8(pitch)
  Virtual Leg to Four Bar/1(back) -> Avoid Hitting Mechanical Limits/1(back_desired)
  Demux4/2 -> Mux11/2
  Demux6/5 -> Virtual Leg to Four Bar/5(dphi)
  Virtual Leg to Four Bar/4(front) -> Avoid Hitting Mechanical Limits/4(front_desired)
  Demux6/6 -> Virtual Leg to Four Bar/6(ddphi)
  Virtual Leg to Four Bar/3(ddback) -> Avoid Hitting Mechanical Limits/3(ddback_desired)
  Virtual Leg to Four Bar/6(ddfront) -> Avoid Hitting Mechanical Limits/6(ddfront_desired)
  Mux11/1 -> Back/Front PD (torque)/5(Measured Velocity [rad/s] [back front])
  Virtual Leg to Four Bar/2(dback) -> Avoid Hitting Mechanical Limits/2(dback_desired)
  Demux6/4 -> Virtual Leg to Four Bar/4(phi)
  Back Motor [rad rad/s]/1 -> Demux5/1
  Demux5/1 -> Mux6/1
  Foot2CoM Z Desired [m m/s m/s^2]/1 -> "Convert CoM (X,Y,Z) to  (Leg Angles, Leg Length)"/3(Z_star)
  Mux4/1 -> Back/Front PD (torque)/2(Desired Velocity [rad/s] [back front])
  Front Motor [rad rad/s]/1 -> Demux4/1
  Demux5/2 -> Mux11/1
  Avoid Hitting Mechanical Limits/3(dback_cmd) -> Mux4/1
  Mux3/1 -> Back/Front PD (torque)/1(Desired Position [rad] [back front])
  Mux6/1 -> Back/Front PD (torque)/4(Measured Position [rad] [back front])
  Avoid Hitting Mechanical Limits/6(ddfront_cmd) -> Mux5/2
  Avoid Hitting Mechanical Limits/5(ddback_cmd) -> Mux5/1
  Avoid Hitting Mechanical Limits/2(front_cmd) -> Mux3/2
  Avoid Hitting Mechanical Limits/4(dfront_cmd) -> Mux4/2
  Avoid Hitting Mechanical Limits/1(back_cmd) -> Mux3/1
  Demux4/1 -> Mux6/2

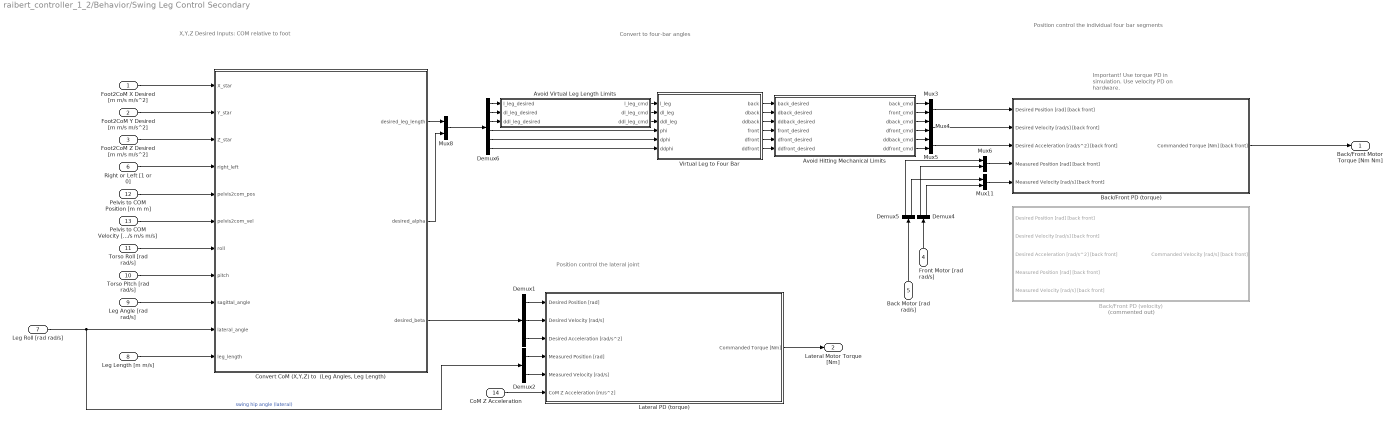
== system raibert_controller_1_2/Behavior/Swing Leg Control Secondary ==
  note: Position control the
      | individual four bar segments
  note: Convert to four-bar angles
  note: X,Y,Z Desired Inputs: COM relative to foot
  note: Important!
      | Use torque PD in simulation.
      | Use velocity PD on hardware.
  note: Position control the lateral joint
  Foot2CoM X Desired [m m/s m/s^2] : Inport
  Foot2CoM Y Desired [m m/s m/s^2] : Inport  Port=2
  Foot2CoM Z Desired [m m/s m/s^2] : Inport  Port=3
  Front Motor [rad rad/s] : Inport  Port=4
  Back Motor [rad rad/s] : Inport  Port=5
  Right or Left [1 or 0] : Inport  Port=6
  Leg Roll [rad rad/s] : Inport  Port=7
  Leg Length [m m/s] : Inport  Port=8
  Leg Angle [rad rad/s] : Inport  Port=9
  Torso Pitch [rad rad/s] : Inport  Port=10
  Torso Roll [rad rad/s] : Inport  Port=11
  Pelvis to COM Position [m m m] : Inport  Port=12
  Pelvis to COM Velocity [m/s m/s m/s] : Inport  Port=13
  CoM Z Acceleration : Inport  Port=14
  Avoid Hitting Mechanical Limits : MATLAB Function  TreatAsAtomicUnit=on
  Avoid Virtual Leg Length Limits : MATLAB Function  TreatAsAtomicUnit=on
  Back/Front PD (torque) : Subsystem
  Back/Front PD (velocity) : Subsystem  Commented=on
  "Convert CoM (X,Y,Z) to  (Leg Angles, Leg Length)" : MATLAB Function  TreatAsAtomicUnit=on
  Demux1 : Demux  Outputs=3
  Demux2 : Demux  Outputs=2
  Demux4 : Demux  Outputs=2
  Demux5 : Demux  Outputs=2
  Demux6 : Demux  Outputs=6
  Lateral PD (torque) : Subsystem
  Mux{3..6,8,11} (6 alike) : Mux  Inputs=2
  Virtual Leg to Four Bar : MATLAB Function  TreatAsAtomicUnit=on
  Back/Front Motor Torque [Nm Nm] : Outport
  Lateral Motor Torque [Nm] : Outport  Port=2
  wires:
  Demux4/1 -> Mux6/2
  Mux6/1 -> Back/Front PD (torque)/4(Measured Position [rad] [back front])
  Mux3/1 -> Back/Front PD (torque)/1(Desired Position [rad] [back front])
  Demux5/2 -> Mux11/1
  Front Motor [rad rad/s]/1 -> Demux4/1
  Mux4/1 -> Back/Front PD (torque)/2(Desired Velocity [rad/s] [back front])
  Foot2CoM Z Desired [m m/s m/s^2]/1 -> "Convert CoM (X,Y,Z) to  (Leg Angles, Leg Length)"/3(Z_star)
  Demux5/1 -> Mux6/1
  Back Motor [rad rad/s]/1 -> Demux5/1
  Demux6/4 -> Virtual Leg to Four Bar/4(phi)
  Mux11/1 -> Back/Front PD (torque)/5(Measured Velocity [rad/s] [back front])
  Demux6/6 -> Virtual Leg to Four Bar/6(ddphi)
  Demux6/5 -> Virtual Leg to Four Bar/5(dphi)
  Demux4/2 -> Mux11/2
  Torso Pitch [rad rad/s]/1 -> "Convert CoM (X,Y,Z) to  (Leg Angles, Leg Length)"/8(pitch)
  Torso Roll [rad rad/s]/1 -> "Convert CoM (X,Y,Z) to  (Leg Angles, Leg Length)"/7(roll)
  Right or Left [1 or 0]/1 -> "Convert CoM (X,Y,Z) to  (Leg Angles, Leg Length)"/4(right_left)
  Leg Roll [rad rad/s]/1 -> Demux2/1, "Convert CoM (X,Y,Z) to  (Leg Angles, Leg Length)"/10(lateral_angle)  "swing hip angle (lateral)"
  Leg Angle [rad rad/s]/1 -> "Convert CoM (X,Y,Z) to  (Leg Angles, Leg Length)"/9(sagittal_angle)
  "Convert CoM (X,Y,Z) to  (Leg Angles, Leg Length)"/2(desired_alpha) -> Mux8/2
  Leg Length [m m/s]/1 -> "Convert CoM (X,Y,Z) to  (Leg Angles, Leg Length)"/11(leg_length)
  "Convert CoM (X,Y,Z) to  (Leg Angles, Leg Length)"/1(desired_leg_length) -> Mux8/1
  Mux8/1 -> Demux6/1
  Foot2CoM Y Desired [m m/s m/s^2]/1 -> "Convert CoM (X,Y,Z) to  (Leg Angles, Leg Length)"/2(Y_star)
  Pelvis to COM Position [m m m]/1 -> "Convert CoM (X,Y,Z) to  (Leg Angles, Leg Length)"/5(pelvis2com_pos)
  Pelvis to COM Velocity [m/s m/s m/s]/1 -> "Convert CoM (X,Y,Z) to  (Leg Angles, Leg Length)"/6(pelvis2com_vel)
  "Convert CoM (X,Y,Z) to  (Leg Angles, Leg Length)"/3(desired_beta) -> Demux1/1
  Back/Front PD (torque)/1(Commanded Torque [Nm] [back front]) -> Back/Front Motor Torque [Nm Nm]/1
  Foot2CoM X Desired [m m/s m/s^2]/1 -> "Convert CoM (X,Y,Z) to  (Leg Angles, Leg Length)"/1(X_star)
  Mux5/1 -> Back/Front PD (torque)/3(Desired Acceleration [rad/s^2] [back front])
  Demux1/1 -> Lateral PD (torque)/1(Desired Position [rad])
  Demux1/3 -> Lateral PD (torque)/3(Desired Acceleration [rad/s^2])
  Demux1/2 -> Lateral PD (torque)/2(Desired Velocity [rad/s])
  Lateral PD (torque)/1(Commanded Torque [Nm]) -> Lateral Motor Torque [Nm]/1
  Demux2/2 -> Lateral PD (torque)/5(Measured Velocity [rad/s])
  Demux2/1 -> Lateral PD (torque)/4(Measured Position [rad])
  CoM Z Acceleration/1 -> Lateral PD (torque)/6(CoM Z Acceleration [m/s^2])
  Virtual Leg to Four Bar/1(back) -> Avoid Hitting Mechanical Limits/1(back_desired)
  Virtual Leg to Four Bar/2(dback) -> Avoid Hitting Mechanical Limits/2(dback_desired)
  Virtual Leg to Four Bar/3(ddback) -> Avoid Hitting Mechanical Limits/3(ddback_desired)
  Virtual Leg to Four Bar/4(front) -> Avoid Hitting Mechanical Limits/4(front_desired)
  Virtual Leg to Four Bar/5(dfront) -> Avoid Hitting Mechanical Limits/5(dfront_desired)
  Virtual Leg to Four Bar/6(ddfront) -> Avoid Hitting Mechanical Limits/6(ddfront_desired)
  Avoid Hitting Mechanical Limits/1(back_cmd) -> Mux3/1
  Avoid Hitting Mechanical Limits/6(ddfront_cmd) -> Mux5/2
  Avoid Hitting Mechanical Limits/2(front_cmd) -> Mux3/2
  Avoid Hitting Mechanical Limits/3(dback_cmd) -> Mux4/1
  Avoid Hitting Mechanical Limits/4(dfront_cmd) -> Mux4/2
  Avoid Hitting Mechanical Limits/5(ddback_cmd) -> Mux5/1
  Demux6/1 -> Avoid Virtual Leg Length Limits/1(l_leg_desired)
  Demux6/2 -> Avoid Virtual Leg Length Limits/2(dl_leg_desired)
  Demux6/3 -> Avoid Virtual Leg Length Limits/3(ddl_leg_desired)
  Avoid Virtual Leg Length Limits/1(l_leg_cmd) -> Virtual Leg to Four Bar/1(l_leg)
  Avoid Virtual Leg Length Limits/2(dl_leg_cmd) -> Virtual Leg to Four Bar/2(dl_leg)
  Avoid Virtual Leg Length Limits/3(ddl_leg_cmd) -> Virtual Leg to Four Bar/3(ddl_leg)
